simulink model "DegradationParameterGenerator"  (R2021a)
settings: Solver=VariableStepAuto  StartTime=0.0  StopTime=10.0  RelTol=1e-3
values from neighbouring files (symbols this model uses):
  gen_P_Fe_Nom_adjustment = 0.5    [Run_GeneratorRectifierBoostConverterInverterMotorModel.m]    (also in Run_GeneratorRectifierBoostConverterModel.m; Run_GeneratorRectifierBuckConverterModel.m; Run_GeneratorRectifierModel.m)
  gen_R_s_adjustment = 0.5    [Run_GeneratorRectifierBoostConverterInverterMotorModel.m]    (also in Run_GeneratorRectifierBoostConverterModel.m; Run_GeneratorRectifierBuckConverterModel.m; Run_GeneratorRectifierModel.m)
undefined symbols (not defined in the file or in its folder): gen_flux_m_adjustment
libraries: Lib_EMTAT x4
settings Model: Creator=sfaulk  LastModifiedBy=mebell

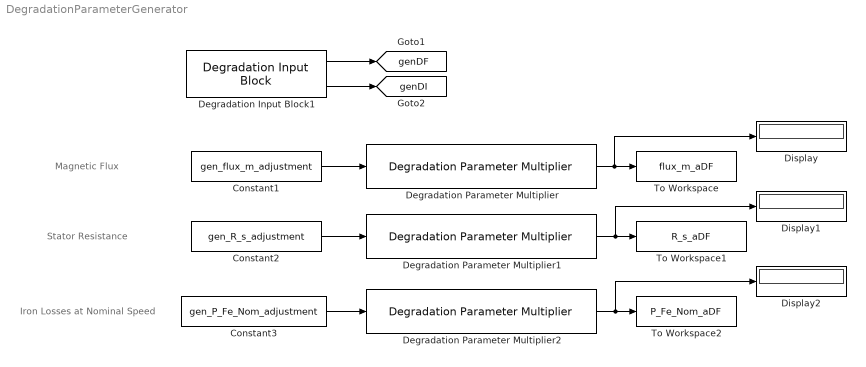
== system DegradationParameterGenerator ==
  note: Stator Resistance
  note: Magnetic Flux
  note: Iron Losses at Nominal Speed
  Constant1 : Constant  Value=gen_flux_m_adjustment
  Constant2 : Constant  Value=gen_R_s_adjustment
  Constant3 : Constant  Value=gen_P_Fe_Nom_adjustment
  Degradation Input Block1 : Lib_EMTAT/Components/Physics-Based/Degradation Input Block  SystemSampleTime=-1  VariantActivationTime=update diagram  Latency=0  AutoFrameSizeCalculation=off
      settings: SourceProductName=EMTAT
  Degradation Parameter Multiplier : Lib_EMTAT/Components/Physics-Based/Degradation Parameter Multiplier  SystemSampleTime=-1  VariantActivationTime=update diagram  Latency=0  AutoFrameSizeCalculation=off
      settings: SourceProductName=EMTAT
  Degradation Parameter Multiplier1 : Lib_EMTAT/Components/Physics-Based/Degradation Parameter Multiplier  SystemSampleTime=-1  VariantActivationTime=update diagram  Latency=0  AutoFrameSizeCalculation=off
      settings: SourceProductName=EMTAT
  Degradation Parameter Multiplier2 : Lib_EMTAT/Components/Physics-Based/Degradation Parameter Multiplier  SystemSampleTime=-1  VariantActivationTime=update diagram  Latency=0  AutoFrameSizeCalculation=off
      settings: SourceProductName=EMTAT
  Display : Display
  Display1 : Display
  Display2 : Display
  To Workspace : ToWorkspace  VariableName=flux_m_aDF  SaveFormat=Timeseries  SampleTime=-1
      settings: Save2DSignal=2-D array (concatenate along first dimension)
  To Workspace1 : ToWorkspace  VariableName=R_s_aDF  SaveFormat=Timeseries  SampleTime=-1
      settings: Save2DSignal=2-D array (concatenate along first dimension)
  To Workspace2 : ToWorkspace  VariableName=P_Fe_Nom_aDF  SaveFormat=Timeseries  SampleTime=-1
      settings: Save2DSignal=2-D array (concatenate along first dimension)
  tag scope: genDF=global, genDI=global
  wires:
  Constant1/1 -> Degradation Parameter Multiplier/1
  Degradation Parameter Multiplier/1 -> Display/1, To Workspace/1
  Degradation Input Block1/2 -> [genDI]
  Degradation Input Block1/1 -> [genDF]
  Degradation Parameter Multiplier1/1 -> Display1/1, To Workspace1/1
  Constant2/1 -> Degradation Parameter Multiplier1/1
  Degradation Parameter Multiplier2/1 -> Display2/1, To Workspace2/1
  Constant3/1 -> Degradation Parameter Multiplier2/1
